simulink model "ex18impcppdcon"  (R2025b)
settings: Solver=VariableStepAuto  StartTime=0.0  StopTime=396  RelTol=1e-3
values from neighbouring files (symbols this model uses):
  IJ = inv(J)    [ex15.m]    (also in ex18.m; ex24.m; ex4.m; ex42.m)
  J = diag([70000, 5900, 9600])    [ex15.m]    (also in ex18.m = diag([7000,5900,9600]); ex19.m = jacobian(f,[x1,x2]); ex24.m = diag([10400, 8200, 9200]); ex4.m = diag([7300, 7000, 3800]))
  q0 = [1;0;0;0]    [ex15.m]    (also in ex18.m; ex24.m = [0.68438, -0.56827,-0.10002,-0.44574]'; ex4.m; ex42.m)
  qr = [-0.06845, -0.5572, 0.8257, -0.05345]'    [ex15.m]    (also in ex18.m = [-.068456,-.55729,0.82576,-.053478]'; ex4.m = [-0.57352, 0.2597, -0.17056, 0.75798]'; ex42.m = [-0.068456,-0.55729,0.82576,-0.053478]')
  w0 = [0;0;0]    [ex15.m]    (also in ex18.m; ex24.m; ex4.m; ex42.m)
libraries: vrlib x1
settings Model: Creator=Esteban  LastModifiedBy=Esteban

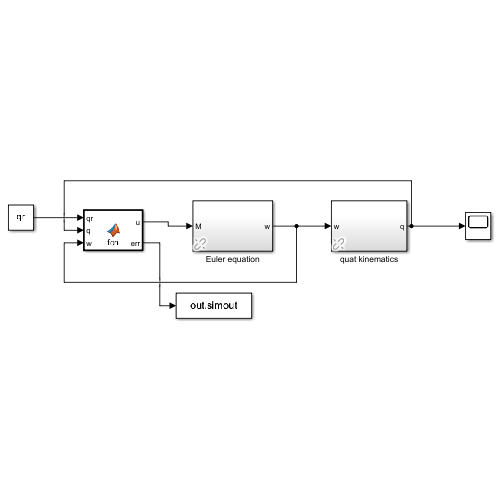
[thumbnail: Simulink's stored preview of the top-level diagram]
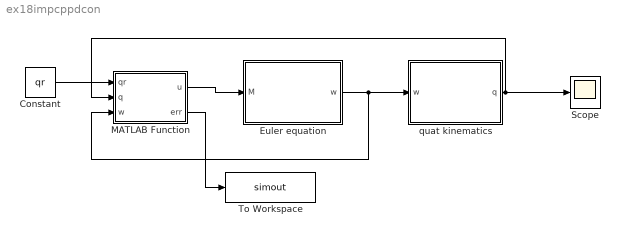
== system ex18impcppdcon ==
  Constant : Constant  Value=qr
  Euler equation : Subsystem  AncestorBlock=lib_rotations_2014/Euler equation
  MATLAB Function : MATLAB Function  TreatAsAtomicUnit=on
  Scope : Scope
  To Workspace : ToWorkspace  VariableName=simout  SaveFormat=Timeseries  SampleTime=-1
  quat kinematics : Subsystem  AncestorBlock=lib_rotations_2014/quat kinematics
  wires:
  MATLAB Function/1(u) -> Euler equation/1(M)
  Euler equation/1(w) -> MATLAB Function/3(w), quat kinematics/1(w)
  quat kinematics/1(q) -> MATLAB Function/2(q), Scope/1
  Constant/1 -> MATLAB Function/1(qr)
  MATLAB Function/2(err) -> To Workspace/1

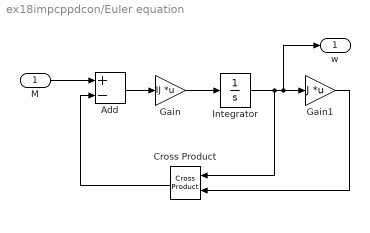
== system ex18impcppdcon/Euler equation ==
  M : Inport
  Add : Sum  Inputs=+-
  Cross Product : vrlib/Utilities/Cross Product
  Gain : Gain  Gain=IJ  Multiplication=Matrix(K*u)
  Gain1 : Gain  Gain=J  Multiplication=Matrix(K*u)
  Integrator : Integrator  InitialCondition=w0
  w : Outport  VectorParamsAs1DForOutWhenUnconnected=off
  wires:
  Cross Product/1 -> Add/2
  Add/1 -> Gain/1
  Gain1/1 -> Cross Product/2
  Gain/1 -> Integrator/1
  Integrator/1 -> Gain1/1, w/1, Cross Product/1
  M/1 -> Add/1

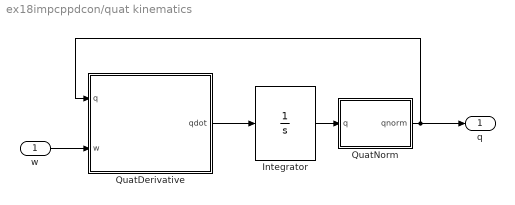
== system ex18impcppdcon/quat kinematics ==
  w : Inport  PortDimensions=3
  Integrator : Integrator  InitialCondition=q0
  QuatDerivative : MATLAB Function  TreatAsAtomicUnit=on
  QuatNorm : MATLAB Function  TreatAsAtomicUnit=on
  q : Outport  PortDimensions=4  VectorParamsAs1DForOutWhenUnconnected=off
  wires:
  w/1 -> QuatDerivative/2(w)
  QuatDerivative/1(qdot) -> Integrator/1
  QuatNorm/1(qnorm) -> QuatDerivative/1(q), q/1
  Integrator/1 -> QuatNorm/1(q)

== matlab function ex18impcppdcon/quat kinematics/QuatDerivative ==
  data: q input; qdot output; w input
function qdot= QuatDerivative(q,w)
%#codegen
omegaq=[0; w];
Q=[q(1) -q(2) -q(3) -q(4);
    q(2) q(1) -q(4) q(3);
    q(3) q(4) q(1) -q(2);
    q(4) -q(3) q(2) q(1)];
qdot=Q*omegaq/2;

== matlab function ex18impcppdcon/quat kinematics/QuatNorm ==
  data: q input; qnorm output
function qnorm = QuatNorm(q)
%#codegen
qnorm=zeros(4,1);
q2=sqrt(q'*q);
qnorm=q/q2;

== matlab function ex18impcppdcon/MATLAB Function ==
  data: qr input; u output; q input; w input; err output
function [u,err] = fcn(qr,q,w)

k1 = 22;
k2 = 196;

qs = [q(1);-q(2:4)];
dq = quatprod(qs,qr);

err = norm(dq(2:4));

u = k1*dq(2:4)-k2*w;
